simulink model "CruiseCtrl"  (R2019b)
settings: Solver=ode45  StartTime=0.0  StopTime=120  RelTol=1e-3
model workspace (MAT data in the model file):
  b = Simulink.Parameter
  b.Value = 50
  b.DataType = 'auto'
  b.Dimensions = [1 1]
  m = Simulink.Parameter
  m.Value = 1000
  m.DataType = 'auto'
  m.Dimensions = [1 1]
  u = Simulink.Parameter
  u.Value = 500
  u.DataType = 'auto'
  u.Dimensions = [1 1]
values from neighbouring files (symbols this model uses):
  b = 50.0    [Var.sldd]
  m = 1000.0    [Var.sldd]
settings Model: Creator=ip  LastModifiedBy=ip

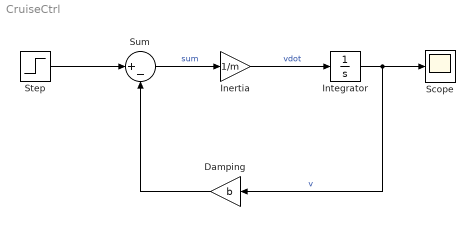
== system CruiseCtrl ==
  Damping : Gain  Gain=b
  Inertia : Gain  Gain=1/m
  Integrator : Integrator
  Scope : Scope
  Step : Step  Time=0  After=u  SampleTime=0
  Sum : Sum  Inputs=|+-
  wires:
  Integrator/1 -> Scope/1, Damping/1  "v"
  Inertia/1 -> Integrator/1  "vdot"
  Sum/1 -> Inertia/1  "sum"
  Damping/1 -> Sum/2
  Step/1 -> Sum/1
